simulink model "partial_pressure_water"  (R2013b)
settings: Solver=ode45  StartTime=0.0  StopTime=10.0  RelTol=1e-3
libraries: carnot x2
settings Model: Creator=drhf  LastModifiedBy=drhf
settings OptimizationCC: InlineParams=on

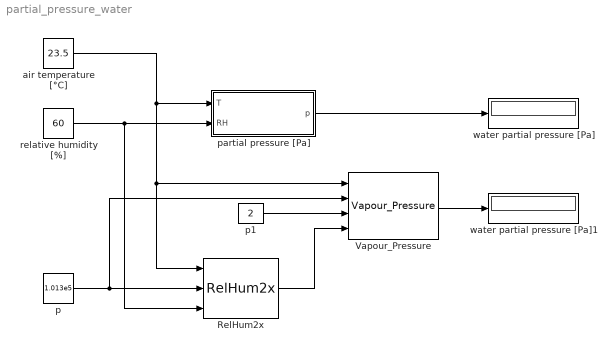
== system partial_pressure_water ==
  RelHum2x : carnot/Basic/Material_Properties/RelHum2x
  Vapour_Pressure : carnot/Basic/Material_Properties/Vapour_Pressure  VariantControl=CarlibClassic  INPUTARGUMENTS=state variables (classic)  DEBUGLEVEL=WARNINGLEVEL  MAXTOTALMESSAGES=inf  MAXCONSECUTIVEMESSAGES=inf  WRITETOFILE=0  FILENAME='errors.txt'
  air temperature [°C] : Constant  Value=23.5
  p : Constant  Value=1.013e5
  p1 : Constant  Value=2
  partial pressure [Pa] : Subsystem
  relative humidity [%] : Constant  Value=60
  water partial pressure [Pa] : Display
  water partial pressure [Pa]1 : Display
  wires:
  air temperature [°C]/1 -> Vapour_Pressure/1, RelHum2x/1, partial pressure [Pa]/1(T)
  relative humidity [%]/1 -> RelHum2x/3, partial pressure [Pa]/2(RH)
  partial pressure [Pa]/1(p) -> water partial pressure [Pa]/1
  p/1 -> Vapour_Pressure/2, RelHum2x/2
  RelHum2x/1 -> Vapour_Pressure/4
  p1/1 -> Vapour_Pressure/3
  Vapour_Pressure/1 -> water partial pressure [Pa]1/1

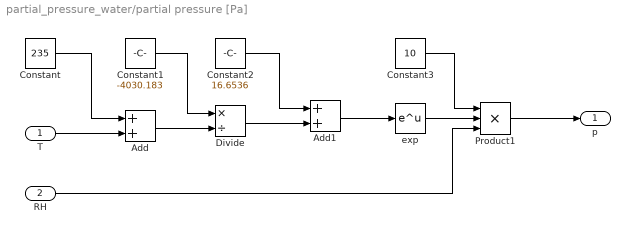
== system partial_pressure_water/partial pressure [Pa] ==
  T : Inport
  RH : Inport  Port=2
  Add : Sum
  Add1 : Sum
  Constant : Constant  Value=235
  Constant1 : Constant  Value=-4030.183
  Constant2 : Constant  Value=16.6536
  Constant3 : Constant  Value=10
  Divide : Product  Inputs=*/
  Product1 : Product  Inputs=3
  exp : Math  SaturateOnIntegerOverflow=on
  p : Outport
  wires:
  Constant/1 -> Add/1
  T/1 -> Add/2
  Add/1 -> Divide/2
  Constant1/1 -> Divide/1
  Divide/1 -> Add1/2
  Constant2/1 -> Add1/1
  Add1/1 -> exp/1
  exp/1 -> Product1/2
  RH/1 -> Product1/3
  Constant3/1 -> Product1/1
  Product1/1 -> p/1
